simulink model "ejercicio3_solve_slx"  (R2024a)
settings: Solver=ode4  StartTime=0.0  StopTime=3*pi  FixedStep=0.01  RelTol=1e-3
settings Model: Creator=pablo  LastModifiedBy=pablo

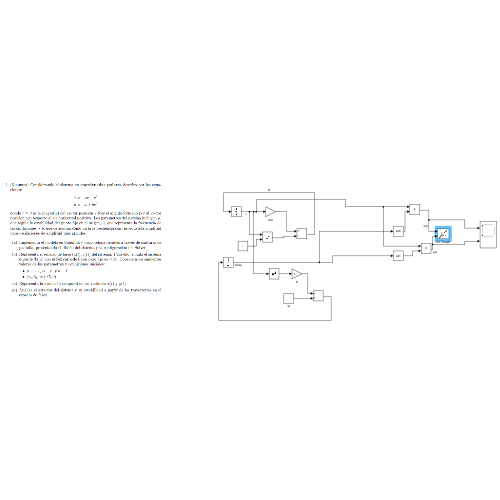
[thumbnail: Simulink's stored preview of the top-level diagram]
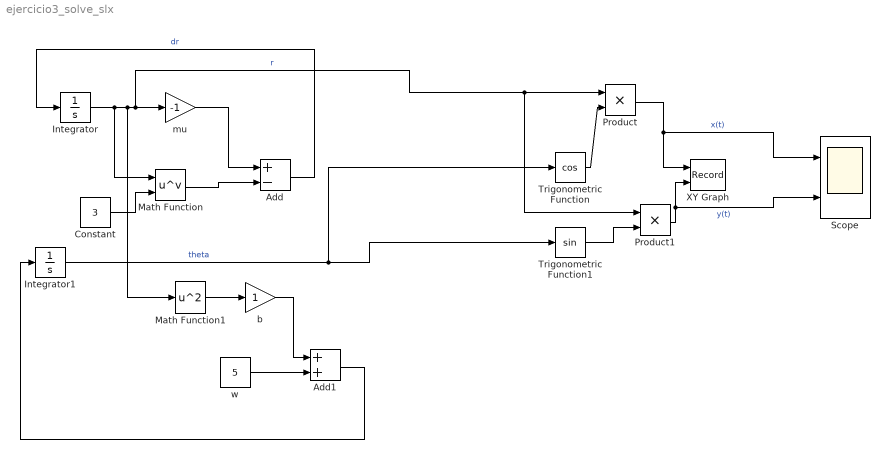
== system ejercicio3_solve_slx ==
  Add : Sum  Inputs=+-
  Add1 : Sum
  Constant : Constant  Value=3
  Integrator : Integrator  InitialCondition=0.5
  Integrator1 : Integrator
  Math Function : Math  Operator=pow
  Math Function1 : Math  Operator=square
  Product : Product
  Product1 : Product
  Scope : Scope  NumInputPorts=2
  Trigonometric Function : Trigonometry  Operator=cos
  Trigonometric Function1 : Trigonometry
  XY Graph : Record  FileSettingsInternal="{\"entries\":[{\"content\":{\"excelSettings\":{\"content\":{},\"type\":\"Streamout.ExcelSettings\"}},\"type\":\"Streamout.FileSettingStorage\",\"uuid\":\"\"}],\"packageUris\":[\"http:\\/\\/schema.mathworks.com\\/mf0\\/streamout_blocks\\/R2020a\"],\"version\":\"1.0\"}"  Layout=[1 1]  SignalsInternal="{\"entries\":[{\"content\":{\"signals\":[{\"content\":{\"blockPath\":[],\"dimensions\":[1],\"domain\":\"\",\"lineColor\":\"#a2142f\",\"plots\":[ 1 ],\"port\":1,\"sid\":[\"\"],\"signalID\":1,\"signalName\":\"x(t)\"},\"type\":\"RecordBlkView.Signal\",\"uuid\":\"\"},{\"content\":{\"blockPath\":[],\"dimensions\":[1],\"domain\":\"\",\"lineColor\":\"#139fff\",\"plots\":[ 1 ],\"port\":2,\"sid\":[\"\"],\"signalID\":2,\"signalName\":\"y(t)\"},\"type\":\"RecordBlkView.Signal\",\"uuid\":\"\"}]},\"type\":\"RecordBlkView.InputSignals\",\"uuid\":\"\"}],\"packageUris\":[\"http:\\/\\/schema.mathworks.com\\/mf0\\/streamout_blocks\\/R2020a\"],\"version\":\"1.0\"}"  VisualizationBindings="{\"xyplotplugin\":{\"info\":[{\"series\":[{\"bindingParametersList\":[{\"parameter\":\"X-Axis\",\"signalID\":1,\"signalName\":\"x(t)\"},{\"parameter\":\"Y-Axis\",\"signalID\":2,\"signalName\":\"y(t)\"},{\"parameter\":\"X-Axis\",\"signalID\":1,\"signalName\":\"x(t)\"},{\"parameter\":\"Y-Axis\",\"signalID\":2,\"signalName\":\"y(t)\"},{\"parameter\":\"X-Axis\",\"signalID\":1,\"signalName\":\"x(t)\"},{\"parameter\":\"Y-Axis\",\"signalID\":2,\"signalName\":\"y(t)\"},{\"parameter\":\"X-Axis\",\"signalID\":1,\"signalName\":\"x(t)\"},{\"parameter\":\"Y-Axis\",\"signalID\":2,\"signalName\":\"y(t)\"}],\"seriesID\":0}],\"subplotID\":1}]}}"  CompatibilityTag=XY
  b : Gain
  mu : Gain  Gain=-1
  w : Constant  Value=5
  wires:
  Integrator/1 -> Math Function1/1, Product/1, Product1/1, mu/1, Math Function/1  "r"
  Constant/1 -> Math Function/2
  Math Function/1 -> Add/2
  mu/1 -> Add/1
  Add/1 -> Integrator/1  "dr"
  w/1 -> Add1/2
  Math Function1/1 -> b/1
  b/1 -> Add1/1
  Add1/1 -> Integrator1/1
  Integrator1/1 -> Trigonometric Function/1, Trigonometric Function1/1  "theta"
  Trigonometric Function/1 -> Product/2
  Product/1 -> Scope/1, XY Graph/1  "x(t)"
  Trigonometric Function1/1 -> Product1/2
  Product1/1 -> Scope/2, XY Graph/2  "y(t)"
